simulink model "tqdtqr_rebuild_V3"  (R2021b)
settings: Solver=VariableStepAuto  StartTime=0.0  StopTime=10.0  RelTol=1e-3
undefined symbols (not defined in the file): ATQD_AfterTqMinGain_X_Deg, ATQD_APSCreepBaseTqD_X_kph, ATQD_APSCreepBaseTqD_Y_Deg, ATQD_APSCreepBaseTqR_X_kph, ATQD_APSCreepBaseTqR_Y_Deg, ATQD_APSCreepIterm_X_kph, ATQD_APSCreepIterm_Y_kph, ATQD_APSCreepPterm_X_kph, ATQD_APSCreepPterm_Y_kph, ATQD_APSDecReq_X_kph, ATQD_APSDecReq_Y_mps2, ATQD_APSDecReqCMD_X_kph, ATQD_APSDecReqTs_X_pct, ATQD_APSDecTimeGain_X_Deg, ATQD_APSDecTimeGain_Y_s, ATQD_APSReqLowSpd_X_Deg, ATQD_AutoHoldReleaseBPS_X_Deg, ATQD_AWDLoadTrqnsGain_X_kg, ATQD_AWDLoadTrqnsGain_Y_pct, ATQD_BOSEnBPSPosn_X_kph, ATQD_BOSMap_X_rpm, ATQD_BOSMap_Y_pct, ATQD_CreepBaseTqD_X_kph, ATQD_CreepBaseTqD_Y_Deg, ATQD_CreepBaseTqR_X_kph, ATQD_CreepBaseTqR_Y_Deg, ATQD_CreepBPSDisPosn_X_Deg, ATQD_CreepBPSDisPosnR_X_Deg, ATQD_CreepBPSEnPosn_X_Deg, ATQD_CreepBPSEnPosnR_X_Deg, ATQD_CreepDeltaTq_X_kph, ATQD_CreepIterm_X_kph, ATQD_CreepIterm_Y_kph, ATQD_CreepItermMaxLimit_X_pct, ATQD_CreepPreloadTime_X_kph, ATQD_CreepPreloadTq_X_kph, ATQD_CreepPreloadTq_Y_s, ATQD_CreepProtTq_X_Deg, ATQD_CreepPterm_X_kph, ATQD_CreepPterm_Y_kph, ATQD_CreepRrTqSpRat_X_rpm, ATQD_CreepRrTqSpRat_Y_Nm, ATQD_CreepTargetSpdD_X_pct, ATQD_CreepTargetSpdR_X_pct, ATQD_CreepUpLimitTq_X_rpm, ATQD_DecIneOPDHoldEnDelay_X_Deg, ATQD_DecIneOPDHoldEnDelay_Y_bar, ATQD_ECOTqMapD_X_rpm, ATQD_ECOTqMapD_Y_pct, ATQD_EMTqMapD_X_rpm, ATQD_EMTqMapD_Y_pct, ATQD_EOPDTqMapDCon_X_rpm, ATQD_EOPDTqMapDCon_Y_Deg, ATQD_EstInitVehWeight_X_c, ATQD_FAfterTqCMDGain_X_rpm, ATQD_FAfterTqCMDGain_Y_pct, ATQD_ForceLowSpd_X_Deg, ATQD_ForcePLimitSpd_X_Deg, ATQD_FrLossMAPLowV_X_rpm, ATQD_FrLossMAPLowV_Y_Nm ... (+949)
libraries: simulink x235, hcu_lib x208, tqr x63, tqd x6
(part 1 of 37)
settings Model: Creator=FVT24123  LastModifiedBy=FVT24123

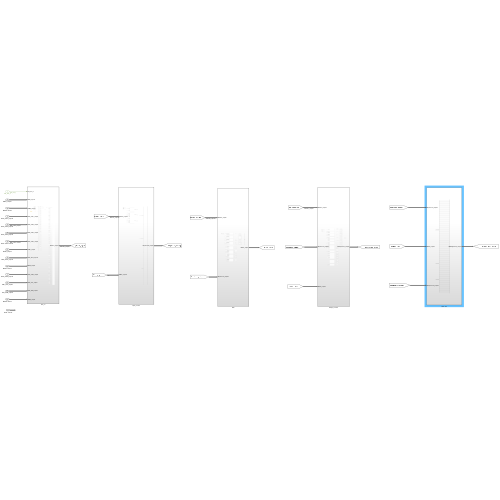
[thumbnail: Simulink's stored preview of the top-level diagram]
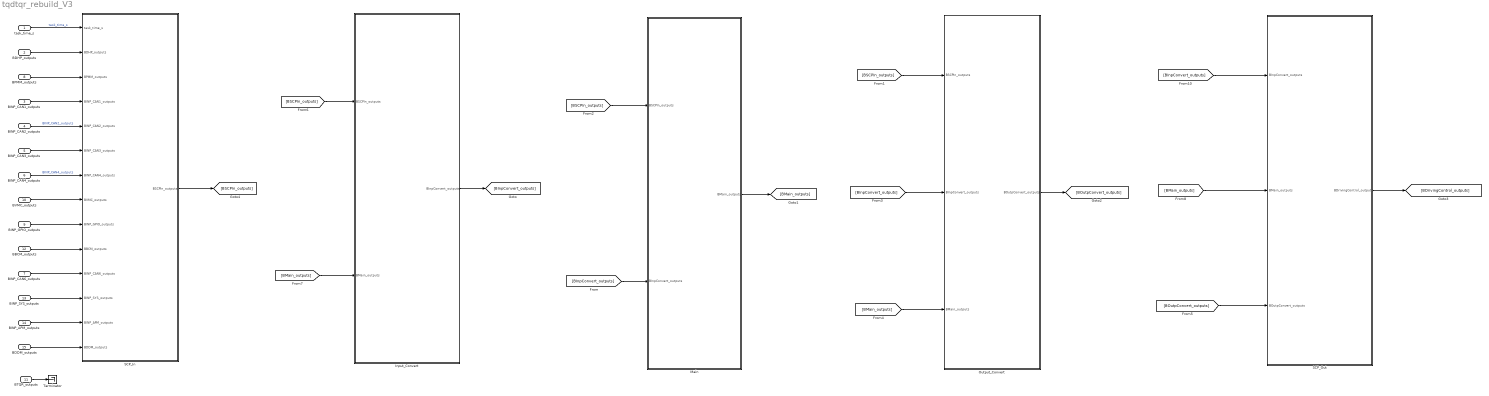
== system tqdtqr_rebuild_V3 ==
  task_time_s : Inport
  BDHP_outputs : Inport  Port=2  OutDataTypeStr=Bus: BDHP_outputs
  BINP_CAN1_outputs : Inport  Port=3  OutDataTypeStr=Bus: BINP_CAN1_outputs
  BINP_CAN2_outputs : Inport  Port=4  OutDataTypeStr=Bus: BINP_CAN2_outputs
  BINP_CAN3_outputs : Inport  Port=5  OutDataTypeStr=Bus: BINP_CAN3_outputs
  BINP_CAN4_outputs : Inport  Port=6  OutDataTypeStr=Bus: BINP_CAN4_outputs
  BINP_CAN6_outputs : Inport  Port=7  OutDataTypeStr=Bus: BINP_CAN6_outputs
  BPMM_outputs : Inport  Port=8  OutDataTypeStr=Bus: BPMM_outputs
  BINP_GPIO_outputs : Inport  Port=9  OutDataTypeStr=Bus: BINP_GPIO_outputs
  BVMC_outputs : Inport  Port=10  OutDataTypeStr=Bus: BVMC_outputs
  BTQR_outputs : Inport  Port=11  OutDataTypeStr=Bus: BTQR_outputs  LockScale=on
  BBCM_outputs : Inport  Port=12  OutDataTypeStr=Bus: BBCM_outputs
  BINP_SYS_outputs : Inport  Port=13  OutDataTypeStr=Bus: BINP_SYS_outputs
  BINP_APM_outputs : Inport  Port=14  OutDataTypeStr=Bus: BINP_APM_outputs
  BDDM_outputs : Inport  Port=15  OutDataTypeStr=Bus: BDDM_outputs
  Input_Convert : Subsystem
  Main : Subsystem
  Output_Convert : Subsystem
  SCP_In : Subsystem
  SCP_Out : Subsystem
  Terminator : Terminator
  wires:
  [BSCPIn_outputs] -> Input_Convert/1(BSCPIn_outputs)
  [BMain_outputs] -> Input_Convert/2(BMain_outputs)
  SCP_In/1(BSCPIn_outputs) -> [BSCPIn_outputs]
  BINP_GPIO_outputs/1 -> SCP_In/9(BINP_GPIO_outputs)
  BTQR_outputs/1 -> Terminator/1
  BINP_SYS_outputs/1 -> SCP_In/12(BINP_SYS_outputs)
  BINP_CAN6_outputs/1 -> SCP_In/11(BINP_CAN6_outputs)
  BDDM_outputs/1 -> SCP_In/14(BDDM_outputs)
  BBCM_outputs/1 -> SCP_In/10(BBCM_outputs)
  BVMC_outputs/1 -> SCP_In/8(BVMC_outputs)
  BDHP_outputs/1 -> SCP_In/2(BDHP_outputs)
  BINP_APM_outputs/1 -> SCP_In/13(BINP_APM_outputs)
  BPMM_outputs/1 -> SCP_In/3(BPMM_outputs)
  BINP_CAN2_outputs/1 -> SCP_In/5(BINP_CAN2_outputs)  "BINP_CAN2_outputs"
  BINP_CAN1_outputs/1 -> SCP_In/4(BINP_CAN1_outputs)
  BINP_CAN4_outputs/1 -> SCP_In/7(BINP_CAN4_outputs)  "BINP_CAN4_outputs"
  task_time_s/1 -> SCP_In/1(task_time_s)  "task_time_s"
  BINP_CAN3_outputs/1 -> SCP_In/6(BINP_CAN3_outputs)
  [BSCPIn_outputs] -> Output_Convert/1(BSCPIn_outputs)
  Input_Convert/1(BInpConvert_outputs) -> [BInpConvert_outputs]
  [BSCPIn_outputs] -> Main/1(BSCPIn_outputs)
  [BInpConvert_outputs] -> Main/2(BInpConvert_outputs)
  Main/1(BMain_outputs) -> [BMain_outputs]
  [BInpConvert_outputs] -> Output_Convert/2(BInpConvert_outputs)
  [BMain_outputs] -> Output_Convert/3(BMain_outputs)
  Output_Convert/1(BOutpConvert_outputs) -> [BOutpConvert_outputs]
  [BInpConvert_outputs] -> SCP_Out/1(BInpConvert_outputs)
  [BMain_outputs] -> SCP_Out/2(BMain_outputs)
  [BOutpConvert_outputs] -> SCP_Out/3(BOutpConvert_outputs)
  SCP_Out/1(BDrivingControl_outputs) -> [BDrivingControl_outputs]

== system tqdtqr_rebuild_V3/Input_Convert ==
  BSCPIn_outputs : Inport
  BMain_outputs : Inport  Port=2
  Bus Creator : BusCreator  Inputs=173
  Bus Selector : BusSelector  OutputSignals=VTQD_LowIdleAccPedal_flg,VTQD_RollRegenDisable_flg,VTQD_BrkSwSta_flg,VTQD_ShiftGearPosn_enum,VTQD_TqTargetShaftSpd_rpm,VTQD_TMRotateDirction_enum,VTQD_EVDriveMode_enum,VTQD_MCUReady4Ext_flg,VTQD_RegenMode_enum,VTQD_FrShaftSpd_rpm,VTQD_RrShaftSpd_rpm,VTQD_LimpHomeAct_flg,VTQD_RDCActive_enum,VTQD_SCPFrRegenAvailTq_Nm,VTQD_SCPRrRegenAvailTq_Nm,VTQD_SCPFrMotorAvailTq_Nm,VTQD_SCPRrMotorAvailTq_Nm,VTQD_SCPFrMCUDCBusVolt_V,VTQD_SCPRrMCUDCBusVolt_V,VTQD_SCPFrMCUTemp_C,VTQD_SCPFrTMTemp_C,VTQD_SCPRrMCUTemp_C,VTQD_SCPRrTMTemp_C,VTQD_SCPSWCRegenUp_flg,VTQD_SCPSWCRegenDown_flg,VTQD_SCPFrEDURotateDirction_enum,VTQD_SCPRrEDURotateDirction_enum,VTQD_SCPFrTMSpd_rpm,VTQD_SCPRrTMSpd_rpm,VTQD_SCPFrEDURealTMTq_Nm,VTQD_SCPRrEDURealTMTq_Nm,VTQD_SCPMCUWarnF_enum,VTQD_SCPMCUWarnR_enum,VTQD_IVIPwrLock_flg,VTQD_IVIPwrLockSta_enum,VTQD_VehActSpd_kph,VTQD_NoSuitbleGear_flg,VTQR_LaunchEn_flg,VTQR_RampTqCMDGain_c,VTQR_EVDriveMode_enum,VTQD_CreepON_flg
  Bus Selector1 : BusSelector  OutputSignals=VTQD_EstVehWeightResult_kg,VTQD_SWCResUpSta_flg,VTQD_SWCSetdownSta_flg,VTQD_SWCCancelSta_flg,SWC_RegenUp,SWC_RegenDown,VTQD_FDCVCURegenMode_enum,VTQD_SaveRegenMode_enum,VTQD_TrailerDisOPDSta_flg,VTQD_SpdCtrlMode_enum,VTQD_SpdCtrlSta_flg,VTQD_SetSpd_kph,VTQD_SWC2ResUpSta_flg,VTQD_SWC2SetdownSta_flg,VTQD_SWC2CancelSta_flg,VTQD_SWC2LADASSta_flg,VTQD_SpdLim4SetSpd_raw32,VTQD_ComboKeyPreEn_flg,VTQD_ComboKeyEn_flg,VTQD_SysMode_enum,VTQD_SWC2ScrollUpSta_flg,VTQD_MaxWhlSlideRate_pct,VTQD_MinWhlSlideRate_pct,VTQD_LeftSlideRate_pct,VTQD_RightSlideRate_pct,VTQD_FrontSlideRate_pct,VTQD_RearSlideRate_pct,VTQD_LFSlideRate_pct,VTQD_LRSlideRate_pct,VTQD_RFSlideRate_pct,VTQD_RRSlideRate_pct,VTQD_SimSouWaveReq_pct,VTQD_SimSoundCmd_pct,VTQD_ActWhlSkipSta_enum,VTQD_SkipDirect_enum,VTQD_GearActualPosn_enum,VTQD_ParkRequest_flg,VTQD_PBWLockTO_flg,VTQD_PBWUnlockTO_flg,VTQD_DriveProtRemove_flg,VTQD_DriveProtEn_flg,VTQD_ForceP_flg,VTQD_DOALatchReq_flg,VTQD_ForcePLimitSpd_kph,VTQD_FrActvDmpDisabReq_flg,VTQD_RrActvDmpDisabReq_flg,VTQD_EPBCarWashMode_flg,VTQD_SWC1SetSpd_kph,VTQD_SWC2SetSpd_kph,VTQD_APSStaSys_enum,VTQD_APSReq_enum,VTQD_APSDecReqA_flg,VTQD_APSDecReq_mps2,VTQD_ActParkRequest_flg,VTQD_APSReqTimer_s,VTQD_OPDHoldEnRel_flg,VTQD_OPDHoldAllowPark_flg,VTQD_OPDHoldLamp_flg,VTQD_OPDHoldActRelTq_Nm,VTQD_OPDHoldDelayForP_flg
  Bus Selector2 : BusSelector  OutputSignals=VTQD_RollRegenEnable_flg,VTQD_BOSEnable_flg,VTQD_BOSTq_Nm,VTQD_IVIRockModeEn_flg,VTQD_LoSpdBrkCtrl_flg,VTQD_RockModeTCSReq_flg,VTQD_RockModePedTq_Nm,VTQD_RockModeTqLim_flg,VTQD_PreLoadPreEn_flg,VTQD_PreloadTq_Nm,VTQD_PreLoadHold_flg,VTQD_CreepWhlTqDem_Nm,VTQD_CreepPrLoadEnable_flg,VTQD_CreepProtTqEn_flg,VTQD_PedalMapWhlTq_Nm,VTQD_EVDriveModeValid_flg,VTQD_RegenTqLimitEn_flg,VTQD_PedAccTqEn_flg,VTQD_SlideRegenLimTq_Nm,VTQD_OPDOn2Off_flg,VTQD_CreepTCSActive_flg,VTQD_FrPreloadTq_Nm,VTQD_RrPreloadTq_Nm,VTQD_CreepEnable_flg,VTQD_CreepBaseTqD_Nm,VTQD_TqSourceFr_enum,VTQD_TqSourceRr_enum,VTQD_TotalWhlTqCapMot_Nm,VTQD_TotalWhlTqCapGen_Nm,VTQD_ForceIdleTqReq_Nm,VTQD_FrEDUSpRat_rat,VTQD_RrEDUSpRat_rat,VTQD_RockModePedTqFr_Nm,VTQD_RockModePedTqRr_Nm,VTQD_TMEnOutpTqSta_enum,VTQD_NewDistFrWhlTq_Nm,VTQD_NewDistRrWhlTq_Nm,VTQD_WhlTqCapMotFr_Nm,VTQD_WhlTqCapMotRr_Nm,VTQD_WhlTqCapGenFr_Nm,VTQD_WhlTqCapGenRr_Nm,VTQD_MotorLossTotal_kW,VTQD_FAfterTqCMDGain_c,VTQD_RAfterTqCMDGain_c,VTQR_FShaftSpdTqLimLow_flg,VTQR_FTimerTqLimLow_flg,VTQR_RShaftSpdTqLimLow_flg,VTQR_RTimerTqLimLow_flg,VTQR_ActFEDUTrqUpLim_Nm,VTQR_ActFEDUTrqLowLim_Nm,VTQR_ActREDUTrqUpLim_Nm,VTQR_ActREDUTrqLowLim_Nm,VTQR_FrTqZeroTransUpBound_Nm,VTQR_FrTqZeroTransLowBound_Nm,VTQR_FrTqZeroTrans_enum,VTQR_RrTqZeroTransUpBound_Nm,VTQR_RrTqZeroTransLowBound_Nm,VTQR_RrTqZeroTrans_enum,VTQR_FrGearChange_flg,VTQR_RrGearChange_flg,VTQR_FrFirstOrderInpTs_c,VTQR_FrRateLimitInc_Nm,VTQR_FrRateLimitDec_Nm,VTQR_RrFirstOrderInpTs_c,VTQR_RrRateLimitInc_Nm,VTQR_RrRateLimitDec_Nm,VTQD_FEDUWhlTqBRegen_Nm,VTQD_REDUWhlTqBRegen_Nm,VTQR_ActFEDUTqLowLimit_Nm,VTQR_ActFEDUTqUpLimit_Nm,VTQR_ActREDUTqUpLimit_Nm,VTQR_ActREDUTqLowLimit_Nm
  Input Signal Convert : Subsystem
  Main function : Subsystem
  Signal function : Subsystem
  BInpConvert_outputs : Outport
  wires:
  BSCPIn_outputs/1 -> [BSCPIn_outputs]
  [BSCPIn_outputs] -> Input Signal Convert/1(BSCPIn_outputs)
  [BSCPIn_outputs] -> Signal function/1(BSCPIn_outputs)
  Input Signal Convert/1(BSignalConvert_outputs) -> [BSignalConvert_outputs]
  [BSignalConvert_outputs] -> Signal function/2(BSignalConvert_outputs)
  [BMain_outputs] -> Signal function/3(BMain_outputs)
  BMain_outputs/1 -> [BMain_outputs]
  [BFunction_outputs] -> Input Signal Convert/2(BFunction_outputs)
  Signal function/1(BFunction_outputs) -> [BFunction_outputs]
  Bus Selector/1 -> Bus Creator/1  "<VTQD_LowIdleAccPedal_flg>"
  Bus Selector/2 -> Bus Creator/2  "<VTQD_RollRegenDisable_flg>"
  Bus Selector/3 -> Bus Creator/3  "<VTQD_BrkSwSta_flg>"
  Bus Selector/4 -> Bus Creator/4  "<VTQD_ShiftGearPosn_enum>"
  Bus Selector/5 -> Bus Creator/5  "<VTQD_TqTargetShaftSpd_rpm>"
  Bus Selector/6 -> Bus Creator/6  "<VTQD_TMRotateDirction_enum>"
  Bus Selector/7 -> Bus Creator/7  "<VTQD_EVDriveMode_enum>"
  Bus Selector/8 -> Bus Creator/8  "<VTQD_MCUReady4Ext_flg>"
  Bus Selector/9 -> Bus Creator/9  "<VTQD_RegenMode_enum>"
  Bus Selector/10 -> Bus Creator/10  "<VTQD_FrShaftSpd_rpm>"
  Bus Selector/11 -> Bus Creator/11  "<VTQD_RrShaftSpd_rpm>"
  Bus Selector/12 -> Bus Creator/12  "<VTQD_LimpHomeAct_flg>"
  Bus Selector/13 -> Bus Creator/13  "<VTQD_RDCActive_enum>"
  Bus Selector/14 -> Bus Creator/14  "<VTQD_SCPFrRegenAvailTq_Nm>"
  Bus Selector/15 -> Bus Creator/15  "<VTQD_SCPRrRegenAvailTq_Nm>"
  Bus Selector/16 -> Bus Creator/16  "<VTQD_SCPFrMotorAvailTq_Nm>"
  Bus Selector/17 -> Bus Creator/17  "<VTQD_SCPRrMotorAvailTq_Nm>"
  Bus Selector/18 -> Bus Creator/18  "<VTQD_SCPFrMCUDCBusVolt_V>"
  [BFunction_outputs] -> Bus Selector1/1
  Bus Selector/19 -> Bus Creator/19  "<VTQD_SCPRrMCUDCBusVolt_V>"
  Bus Selector/20 -> Bus Creator/20  "<VTQD_SCPFrMCUTemp_C>"
  Bus Selector/21 -> Bus Creator/21  "<VTQD_SCPFrTMTemp_C>"
  Bus Selector/22 -> Bus Creator/22  "<VTQD_SCPRrMCUTemp_C>"
  Bus Selector/23 -> Bus Creator/23  "<VTQD_SCPRrTMTemp_C>"
  Bus Selector/24 -> Bus Creator/24  "<VTQD_SCPSWCRegenUp_flg>"
  Bus Selector/25 -> Bus Creator/25  "<VTQD_SCPSWCRegenDown_flg>"
  Bus Selector/26 -> Bus Creator/26  "<VTQD_SCPFrEDURotateDirction_enum>"
  Bus Selector/27 -> Bus Creator/27  "<VTQD_SCPRrEDURotateDirction_enum>"
  Bus Selector/28 -> Bus Creator/28  "<VTQD_SCPFrTMSpd_rpm>"
  Bus Selector/29 -> Bus Creator/29  "<VTQD_SCPRrTMSpd_rpm>"
  Bus Selector/30 -> Bus Creator/30  "<VTQD_SCPFrEDURealTMTq_Nm>"
  Bus Selector/31 -> Bus Creator/31  "<VTQD_SCPRrEDURealTMTq_Nm>"
  Bus Selector/32 -> Bus Creator/32  "<VTQD_SCPMCUWarnF_enum>"
  Bus Selector/33 -> Bus Creator/33  "<VTQD_SCPMCUWarnR_enum>"
  Bus Selector1/1 -> Bus Creator/42  "<VTQD_EstVehWeightResult_kg>"
  Bus Selector1/2 -> Bus Creator/43  "<VTQD_SWCResUpSta_flg>"
  Bus Selector1/3 -> Bus Creator/44  "<VTQD_SWCSetdownSta_flg>"
  Bus Selector1/4 -> Bus Creator/45  "<VTQD_SWCCancelSta_flg>"
  Bus Selector1/5 -> Bus Creator/46  "<SWC_RegenUp>"
  Bus Selector1/6 -> Bus Creator/47  "<SWC_RegenDown>"
  Bus Selector1/7 -> Bus Creator/48  "<VTQD_FDCVCURegenMode_enum>"
  Bus Selector1/8 -> Bus Creator/49  "<VTQD_SaveRegenMode_enum>"
  Bus Selector1/9 -> Bus Creator/50  "<VTQD_TrailerDisOPDSta_flg>"
  Bus Selector1/10 -> Bus Creator/51  "<VTQD_SpdCtrlMode_enum>"
  Bus Selector1/11 -> Bus Creator/52  "<VTQD_SpdCtrlSta_flg>"
  Bus Selector1/12 -> Bus Creator/53  "<VTQD_SetSpd_kph>"
  Bus Selector1/13 -> Bus Creator/54  "<VTQD_SWC2ResUpSta_flg>"
  Bus Selector1/14 -> Bus Creator/55  "<VTQD_SWC2SetdownSta_flg>"
  Bus Selector1/15 -> Bus Creator/56  "<VTQD_SWC2CancelSta_flg>"
  Bus Selector1/16 -> Bus Creator/57  "<VTQD_SWC2LADASSta_flg>"
  Bus Selector1/17 -> Bus Creator/58  "<VTQD_SpdLim4SetSpd_raw32>"
  Bus Selector1/18 -> Bus Creator/59  "<VTQD_ComboKeyPreEn_flg>"
  Bus Selector1/19 -> Bus Creator/60  "<VTQD_ComboKeyEn_flg>"
  Bus Selector1/20 -> Bus Creator/61  "<VTQD_SysMode_enum>"
  Bus Creator/1 -> BInpConvert_outputs/1
  [BSignalConvert_outputs] -> Bus Selector/1
  Bus Selector1/48 -> Bus Creator/89  "<VTQD_SWC1SetSpd_kph>"
  Bus Selector1/49 -> Bus Creator/90  "<VTQD_SWC2SetSpd_kph>"
  [DriverWhlTqDemFunc_outputs] -> Bus Selector2/1
  Bus Selector2/1 -> Bus Creator/102  "<VTQD_RollRegenEnable_flg>"
  Bus Selector2/2 -> Bus Creator/103  "<VTQD_BOSEnable_flg>"
  Bus Selector2/3 -> Bus Creator/104  "<VTQD_BOSTq_Nm>"
  Bus Selector2/5 -> Bus Creator/106  "<VTQD_LoSpdBrkCtrl_flg>"
  Bus Selector2/7 -> Bus Creator/108  "<VTQD_RockModePedTq_Nm>"
  Bus Selector2/8 -> Bus Creator/109  "<VTQD_RockModeTqLim_flg>"
  Bus Selector2/9 -> Bus Creator/110  "<VTQD_PreLoadPreEn_flg>"
  Bus Selector2/10 -> Bus Creator/111  "<VTQD_PreloadTq_Nm>"
  Bus Selector2/11 -> Bus Creator/112  "<VTQD_PreLoadHold_flg>"
  Bus Selector2/12 -> Bus Creator/113  "<VTQD_CreepWhlTqDem_Nm>"
  Bus Selector2/13 -> Bus Creator/114  "<VTQD_CreepPrLoadEnable_flg>"
  Bus Selector2/14 -> Bus Creator/115  "<VTQD_CreepProtTqEn_flg>"
  Bus Selector2/15 -> Bus Creator/116  "<VTQD_PedalMapWhlTq_Nm>"
  Bus Selector2/16 -> Bus Creator/117  "<VTQD_EVDriveModeValid_flg>"
  Bus Selector2/17 -> Bus Creator/118  "<VTQD_RegenTqLimitEn_flg>"
  Bus Selector2/18 -> Bus Creator/119  "<VTQD_PedAccTqEn_flg>"
  Bus Selector2/19 -> Bus Creator/120  "<VTQD_SlideRegenLimTq_Nm>"
  Bus Selector2/20 -> Bus Creator/121  "<VTQD_OPDOn2Off_flg>"
  Bus Selector2/21 -> Bus Creator/122  "<VTQD_CreepTCSActive_flg>"
  Bus Selector2/22 -> Bus Creator/123  "<VTQD_FrPreloadTq_Nm>"
  Bus Selector/36 -> Bus Creator/36  "<VTQD_VehActSpd_kph>"
  Bus Selector2/23 -> Bus Creator/124  "<VTQD_RrPreloadTq_Nm>"
  Bus Selector2/24 -> Bus Creator/125  "<VTQD_CreepEnable_flg>"
  Bus Selector2/25 -> Bus Creator/126  "<VTQD_CreepBaseTqD_Nm>"
  [BMain_outputs] -> Main function/4(BMain_outputs)
  [BSignalConvert_outputs] -> Main function/2(BSignalConvert_outputs)
  [BSCPIn_outputs] -> Main function/1(BSCPIn_outputs)
  [BFunction_outputs] -> Main function/3(BFunction_outputs)
  Main function/1(MainFunction_outputs) -> [DriverWhlTqDemFunc_outputs]
  Bus Selector/37 -> Bus Creator/37  "<VTQD_NoSuitbleGear_flg>"
  [DriverWhlTqDemFunc_outputs] -> Signal function/4(DriverWhlTqDemFunc_outputs)
  Bus Selector2/4 -> Bus Creator/105  "<VTQD_IVIRockModeEn_flg>"
  Bus Selector2/6 -> Bus Creator/107  "<VTQD_RockModeTCSReq_flg>"
  Bus Selector1/21 -> Bus Creator/62  "<VTQD_SWC2ScrollUpSta_flg>"
  Bus Selector1/22 -> Bus Creator/63  "<VTQD_MaxWhlSlideRate_pct>"
  Bus Selector1/23 -> Bus Creator/64  "<VTQD_MinWhlSlideRate_pct>"
  Bus Selector1/24 -> Bus Creator/65  "<VTQD_LeftSlideRate_pct>"
  Bus Selector1/25 -> Bus Creator/66  "<VTQD_RightSlideRate_pct>"
  Bus Selector1/26 -> Bus Creator/67  "<VTQD_FrontSlideRate_pct>"
  Bus Selector1/27 -> Bus Creator/68  "<VTQD_RearSlideRate_pct>"
  Bus Selector1/28 -> Bus Creator/69  "<VTQD_LFSlideRate_pct>"
  Bus Selector1/29 -> Bus Creator/70  "<VTQD_LRSlideRate_pct>"
  Bus Selector1/30 -> Bus Creator/71  "<VTQD_RFSlideRate_pct>"
  Bus Selector1/31 -> Bus Creator/72  "<VTQD_RRSlideRate_pct>"
  Bus Selector1/32 -> Bus Creator/73  "<VTQD_SimSouWaveReq_pct>"
  Bus Selector1/33 -> Bus Creator/74  "<VTQD_SimSoundCmd_pct>"
  Bus Selector1/34 -> Bus Creator/75  "<VTQD_ActWhlSkipSta_enum>"
  Bus Selector1/35 -> Bus Creator/76  "<VTQD_SkipDirect_enum>"
  Bus Selector1/36 -> Bus Creator/77  "<VTQD_GearActualPosn_enum>"
  Bus Selector1/37 -> Bus Creator/78  "<VTQD_ParkRequest_flg>"
  Bus Selector1/38 -> Bus Creator/79  "<VTQD_PBWLockTO_flg>"
  Bus Selector1/39 -> Bus Creator/80  "<VTQD_PBWUnlockTO_flg>"
  Bus Selector1/40 -> Bus Creator/81  "<VTQD_DriveProtRemove_flg>"
  Bus Selector1/41 -> Bus Creator/82  "<VTQD_DriveProtEn_flg>"
  Bus Selector1/42 -> Bus Creator/83  "<VTQD_ForceP_flg>"
  Bus Selector1/45 -> Bus Creator/86  "<VTQD_FrActvDmpDisabReq_flg>"
  Bus Selector1/46 -> Bus Creator/87  "<VTQD_RrActvDmpDisabReq_flg>"
  Bus Selector1/47 -> Bus Creator/88  "<VTQD_EPBCarWashMode_flg>"
  Bus Selector/34 -> Bus Creator/34  "<VTQD_IVIPwrLock_flg>"
  Bus Selector/35 -> Bus Creator/35  "<VTQD_IVIPwrLockSta_enum>"
  Bus Selector1/60 -> Bus Creator/101  "<VTQD_OPDHoldDelayForP_flg>"
  Bus Selector1/59 -> Bus Creator/100  "<VTQD_OPDHoldActRelTq_Nm>"
  Bus Selector1/58 -> Bus Creator/99  "<VTQD_OPDHoldLamp_flg>"
  Bus Selector1/57 -> Bus Creator/98  "<VTQD_OPDHoldAllowPark_flg>"
  Bus Selector1/56 -> Bus Creator/97  "<VTQD_OPDHoldEnRel_flg>"
  Bus Selector1/55 -> Bus Creator/96  "<VTQD_APSReqTimer_s>"
  Bus Selector1/54 -> Bus Creator/95  "<VTQD_ActParkRequest_flg>"
  Bus Selector1/53 -> Bus Creator/94  "<VTQD_APSDecReq_mps2>"
  Bus Selector1/52 -> Bus Creator/93  "<VTQD_APSDecReqA_flg>"
  Bus Selector1/51 -> Bus Creator/92  "<VTQD_APSReq_enum>"
  Bus Selector1/50 -> Bus Creator/91  "<VTQD_APSStaSys_enum>"
  Bus Selector/38 -> Bus Creator/38  "<VTQR_LaunchEn_flg>"
  Bus Selector/39 -> Bus Creator/39  "<VTQR_RampTqCMDGain_c>"
  Bus Selector/40 -> Bus Creator/40  "<VTQR_EVDriveMode_enum>"
  Bus Selector2/26 -> Bus Creator/127  "<VTQD_TqSourceFr_enum>"
  Bus Selector2/27 -> Bus Creator/128  "<VTQD_TqSourceRr_enum>"
  Bus Selector2/28 -> Bus Creator/129  "<VTQD_TotalWhlTqCapMot_Nm>"
  Bus Selector2/29 -> Bus Creator/130  "<VTQD_TotalWhlTqCapGen_Nm>"
  Bus Selector2/38 -> Bus Creator/139  "<VTQD_WhlTqCapMotFr_Nm>"
  Bus Selector2/39 -> Bus Creator/140  "<VTQD_WhlTqCapMotRr_Nm>"
  Bus Selector2/40 -> Bus Creator/141  "<VTQD_WhlTqCapGenFr_Nm>"
  Bus Selector2/41 -> Bus Creator/142  "<VTQD_WhlTqCapGenRr_Nm>"
  Bus Selector2/42 -> Bus Creator/143  "<VTQD_MotorLossTotal_kW>"
  Bus Selector2/43 -> Bus Creator/144  "<VTQD_FAfterTqCMDGain_c>"
  Bus Selector2/44 -> Bus Creator/145  "<VTQD_RAfterTqCMDGain_c>"
  Bus Selector2/45 -> Bus Creator/146  "<VTQR_FShaftSpdTqLimLow_flg>"
  Bus Selector2/46 -> Bus Creator/147  "<VTQR_FTimerTqLimLow_flg>"
  Bus Selector2/47 -> Bus Creator/148  "<VTQR_RShaftSpdTqLimLow_flg>"
  Bus Selector2/48 -> Bus Creator/149  "<VTQR_RTimerTqLimLow_flg>"
  Bus Selector2/49 -> Bus Creator/150  "<VTQR_ActFEDUTrqUpLim_Nm>"
  Bus Selector2/50 -> Bus Creator/151  "<VTQR_ActFEDUTrqLowLim_Nm>"
  Bus Selector2/51 -> Bus Creator/152  "<VTQR_ActREDUTrqUpLim_Nm>"
  Bus Selector2/52 -> Bus Creator/153  "<VTQR_ActREDUTrqLowLim_Nm>"
  Bus Selector2/53 -> Bus Creator/154  "<VTQR_FrTqZeroTransUpBound_Nm>"
  Bus Selector2/54 -> Bus Creator/155  "<VTQR_FrTqZeroTransLowBound_Nm>"
  Bus Selector2/55 -> Bus Creator/156  "<VTQR_FrTqZeroTrans_enum>"
  Bus Selector2/56 -> Bus Creator/157  "<VTQR_RrTqZeroTransUpBound_Nm>"
  Bus Selector2/57 -> Bus Creator/158  "<VTQR_RrTqZeroTransLowBound_Nm>"
  Bus Selector2/58 -> Bus Creator/159  "<VTQR_RrTqZeroTrans_enum>"
  Bus Selector2/59 -> Bus Creator/160  "<VTQR_FrGearChange_flg>"
  Bus Selector2/60 -> Bus Creator/161  "<VTQR_RrGearChange_flg>"
  Bus Selector2/61 -> Bus Creator/162  "<VTQR_FrFirstOrderInpTs_c>"
  Bus Selector2/62 -> Bus Creator/163  "<VTQR_FrRateLimitInc_Nm>"
  Bus Selector2/63 -> Bus Creator/164  "<VTQR_FrRateLimitDec_Nm>"
  Bus Selector2/64 -> Bus Creator/165  "<VTQR_RrFirstOrderInpTs_c>"
  Bus Selector2/65 -> Bus Creator/166  "<VTQR_RrRateLimitInc_Nm>"
  Bus Selector2/66 -> Bus Creator/167  "<VTQR_RrRateLimitDec_Nm>"
  Bus Selector2/67 -> Bus Creator/168  "<VTQD_FEDUWhlTqBRegen_Nm>"
  Bus Selector2/68 -> Bus Creator/169  "<VTQD_REDUWhlTqBRegen_Nm>"
  Bus Selector2/69 -> Bus Creator/170  "<VTQR_ActFEDUTqLowLimit_Nm>"
  Bus Selector2/70 -> Bus Creator/171  "<VTQR_ActFEDUTqUpLimit_Nm>"
  Bus Selector2/71 -> Bus Creator/172  "<VTQR_ActREDUTqUpLimit_Nm>"
  Bus Selector2/72 -> Bus Creator/173  "<VTQR_ActREDUTqLowLimit_Nm>"
  [BMain_outputs] -> Input Signal Convert/3(BMain_outputs)
  Bus Selector1/43 -> Bus Creator/84  "<VTQD_DOALatchReq_flg>"
  Bus Selector1/44 -> Bus Creator/85  "<VTQD_ForcePLimitSpd_kph>"
  Bus Selector2/30 -> Bus Creator/131  "<VTQD_ForceIdleTqReq_Nm>"
  Bus Selector2/31 -> Bus Creator/132  "<VTQD_FrEDUSpRat_rat>"
  Bus Selector2/32 -> Bus Creator/133  "<VTQD_RrEDUSpRat_rat>"
  Bus Selector2/33 -> Bus Creator/134  "<VTQD_RockModePedTqFr_Nm>"
  Bus Selector2/34 -> Bus Creator/135  "<VTQD_RockModePedTqRr_Nm>"
  Bus Selector2/35 -> Bus Creator/136  "<VTQD_TMEnOutpTqSta_enum>"
  Bus Selector2/36 -> Bus Creator/137  "<VTQD_NewDistFrWhlTq_Nm>"
  Bus Selector2/37 -> Bus Creator/138  "<VTQD_NewDistRrWhlTq_Nm>"
  Bus Selector/41 -> Bus Creator/41  "<VTQD_CreepON_flg>"

== system tqdtqr_rebuild_V3/Main ==
  note: --------------------------------------------------------------------TQR-----------------------------------------------------------------------
  BSCPIn_outputs : Inport
  BInpConvert_outputs : Inport  Port=2
  Avaliable Tq Limit : Subsystem
  Bus Creator : BusCreator  Inputs=22
  DriverWhlTqDem : Subsystem
  Front/Rear final torque : Subsystem
  Front/Rear first order input torque : Subsystem
  Front/Rear ramp enable judge : Subsystem
  Inverse and turn to motor torque : Subsystem
  Tq Coordination : Subsystem
  Tq Distribution : Subsystem
  BMain_outputs : Outport
  wires:
  BSCPIn_outputs/1 -> [BSCPIn_outputs]
  BInpConvert_outputs/1 -> [BInpConvert_outputs]
  [BSCPIn_outputs] -> DriverWhlTqDem/1(BSCPIn_outputs)
  [BInpConvert_outputs] -> DriverWhlTqDem/2(BInpConvert_outputs)
  DriverWhlTqDem/1(VTQD_DriverWhlTqDem_Nm) -> [VTQD_DriverWhlTqDem_Nm]
  [BSCPIn_outputs] -> Tq Coordination/1(BSCPIn_outputs)
  [BInpConvert_outputs] -> Tq Coordination/2(BInpConvert_outputs)
  [VTQD_DriverWhlTqDem_Nm] -> Tq Coordination/3(VTQD_DriverWhlTqDem_Nm)
  [BSCPIn_outputs] -> Tq Distribution/1(BSCPIn_outputs)
  [BInpConvert_outputs] -> Tq Distribution/2(BInpConvert_outputs)
  Tq Coordination/1(VTQD_CoordTqDem_Nm) -> [VTQD_CoordTqDem_Nm]
  [VTQD_CoordTqDem_Nm] -> Tq Distribution/3(TqCoordination_outputs)
  Tq Distribution/1(VTQD_CoordWhlTqDemFr_Nm) -> [VTQD_CoordWhlTqDemFr_Nm]
  [VTQD_DriverWhlTqDem_Nm] -> Bus Creator/1
  [VTQD_CoordTqDem_Nm] -> Bus Creator/2
  Bus Creator/1 -> BMain_outputs/1
  Tq Distribution/2(VTQD_CoordWhlTqDemRr_Nm) -> [VTQD_CoordWhlTqDemRr_Nm]
  [VTQD_CoordWhlTqDemFr_Nm] -> Bus Creator/3
  [BInpConvert_outputs] -> Avaliable Tq Limit/2(BInpConvert_outputs)
  [BSCPIn_outputs] -> Avaliable Tq Limit/1(BSCPIn_outputs)
  [VTQD_CoordWhlTqDemFr_Nm] -> Avaliable Tq Limit/3(VTQD_CoordWhlTqDemFr_Nm)
  [VTQD_CoordWhlTqDemRr_Nm] -> Avaliable Tq Limit/4(VTQD_CoordWhlTqDemRr_Nm)
  Avaliable Tq Limit/2(VTQD_AfterAvailableTqDemRr_Nm) -> [VTQD_AfterAvailableTqDemRr_Nm]
  Avaliable Tq Limit/1(VTQD_AfterAvailableTqDemFr_Nm) -> [VTQD_AfterAvailableTqDemFr_Nm]
  [VTQD_AfterAvailableTqDemFr_Nm] -> Bus Creator/7
  [VTQD_AfterAvailableTqDemRr_Nm] -> Bus Creator/8
  [BInpConvert_outputs] -> Front/Rear first order input torque/1(BInpConvert_outputs)
  [VTQD_AfterAvailableTqDemFr_Nm] -> Front/Rear first order input torque/2(VTQD_AfterAvailableTqDemFr_Nm)
  [VTQD_AfterAvailableTqDemRr_Nm] -> Front/Rear first order input torque/3(VTQD_AfterAvailableTqDemRr_Nm)
  Front/Rear first order input torque/1(VTQR_FrFirstOrderInpTq_Nm) -> [VTQR_FrFirstOrderInpTq_Nm]
  Front/Rear first order input torque/2(VTQR_RrFirstOrderInpTq_Nm) -> [VTQR_RrFirstOrderInpTq_Nm]
  [BInpConvert_outputs] -> Front/Rear final torque/2(BInpConvert_outputs)
  [VTQR_FrFirstOrderInpTq_Nm] -> Front/Rear final torque/3(VTQR_FrFirstOrderInpTq_Nm)
  [VTQR_RrFirstOrderInpTq_Nm] -> Front/Rear final torque/4(VTQR_RrFirstOrderInpTq_Nm)
  [BSCPIn_outputs] -> Front/Rear final torque/1(BSCPIn_outputs)
  Front/Rear final torque/1(VTQR_FrFirstOrderOutTqDelay_Nm) -> [VTQR_FrFirstOrderOutTqDelay_Nm]
  Front/Rear final torque/2(VTQR_FEDUWhlTqReqSmoothDelay_Nm) -> [VTQR_FEDUWhlTqReqSmoothDelay_Nm]
  Front/Rear final torque/3(VTQR_RampFEDUWhlTqReq_Nm) -> [VTQR_RampFEDUWhlTqReq_Nm]
  Front/Rear final torque/4(VTQR_RrFirstOrderOutTqDelay_Nm) -> [VTQR_RrFirstOrderOutTqDelay_Nm]
  Front/Rear final torque/5(VTQR_REDUWhlTqReqSmoothDelay_Nm) -> [VTQR_REDUWhlTqReqSmoothDelay_Nm]
  Front/Rear final torque/6(VTQR_RampREDUWhlTqReq_Nm) -> [VTQR_RampREDUWhlTqReq_Nm]
  [VTQR_FrFirstOrderOutTqDelay_Nm] -> Bus Creator/11
  [VTQR_FEDUWhlTqReqSmoothDelay_Nm] -> Bus Creator/12
  [VTQR_RampFEDUWhlTqReq_Nm] -> Bus Creator/13
  [VTQR_RrFirstOrderOutTqDelay_Nm] -> Bus Creator/14
  [VTQR_REDUWhlTqReqSmoothDelay_Nm] -> Bus Creator/15
  [VTQR_RampREDUWhlTqReq_Nm] -> Bus Creator/16
  [VTQR_FrFirstOrderInpTq_Nm] -> Bus Creator/9
  [VTQR_RrFirstOrderInpTq_Nm] -> Bus Creator/10
  [VTQR_FrFirstOrderOutTqDelay_Nm] -> Front/Rear first order input torque/4(VTQR_FrFirstOrderOutTqDelay_Nm)
  [VTQR_RrFirstOrderOutTqDelay_Nm] -> Front/Rear first order input torque/5(VTQR_RrFirstOrderOutTqDelay_Nm)
  [BSCPIn_outputs] -> Front/Rear ramp enable judge/1(BSCPIn_outputs)
  [BInpConvert_outputs] -> Front/Rear ramp enable judge/2(BInpConvert_outputs)
  [VTQR_RampFEDUWhlTqReq_Nm] -> Front/Rear ramp enable judge/3(VTQR_RampFEDUWhlTqReq_Nm)
  [VTQD_AfterAvailableTqDemFr_Nm] -> Front/Rear ramp enable judge/4(VTQD_AfterAvailableTqDemFr_Nm)
  [VTQR_RampREDUWhlTqReq_Nm] -> Front/Rear ramp enable judge/5(VTQR_RampREDUWhlTqReq_Nm)
  [VTQD_AfterAvailableTqDemRr_Nm] -> Front/Rear ramp enable judge/6(VTQD_AfterAvailableTqDemRr_Nm)
  Front/Rear ramp enable judge/1(VTQR_ActualFEDUWhlTqReq_Nm) -> [VTQR_ActualFEDUWhlTqReq_Nm]
  Front/Rear ramp enable judge/2(VTQR_NoABSFEDUWhlTqReq_Nm) -> [VTQR_NoABSFEDUWhlTqReq_Nm]
  Front/Rear ramp enable judge/3(VTQR_ActualREDUWhlTqReq_Nm) -> [VTQR_ActualREDUWhlTqReq_Nm]
  Front/Rear ramp enable judge/4(VTQR_NoABSREDUWhlTqReq_Nm) -> [VTQR_NoABSREDUWhlTqReq_Nm]
  [VTQR_ActualFEDUWhlTqReq_Nm] -> Bus Creator/17
  [VTQR_NoABSFEDUWhlTqReq_Nm] -> Bus Creator/18
  [VTQR_ActualREDUWhlTqReq_Nm] -> Bus Creator/19
  [VTQR_NoABSREDUWhlTqReq_Nm] -> Bus Creator/20
  [BSCPIn_outputs] -> Inverse and turn to motor torque/1(BSCPIn_outputs)
  [BInpConvert_outputs] -> Inverse and turn to motor torque/2(BInpConvert_outputs)
  [VTQR_ActualFEDUWhlTqReq_Nm] -> Inverse and turn to motor torque/3(VTQR_ActualFEDUWhlTqReq_Nm)
  [VTQR_ActualREDUWhlTqReq_Nm] -> Inverse and turn to motor torque/4(VTQR_ActualREDUWhlTqReq_Nm)
  Inverse and turn to motor torque/1(VTQR_FrTMTqReq_Nm) -> [VTQR_FrTMTqReq_Nm]
  Inverse and turn to motor torque/2(VTQR_RrTMTqReq_Nm) -> [VTQR_RrTMTqReq_Nm]
  [VTQR_FrTMTqReq_Nm] -> Bus Creator/21
  [VTQR_RrTMTqReq_Nm] -> Bus Creator/22
  Tq Distribution/3(VTQD_CoordTqDemFr_Nm) -> [VTQD_CoordTqDemFr_Nm]
  Tq Distribution/4(VTQD_CoordTqDemRr_Nm) -> [VTQD_CoordTqDemRr_Nm]
  [VTQD_CoordWhlTqDemRr_Nm] -> Bus Creator/4
  [VTQD_CoordTqDemFr_Nm] -> Bus Creator/5
  [VTQD_CoordTqDemRr_Nm] -> Bus Creator/6

== system tqdtqr_rebuild_V3/Output_Convert ==
  BSCPIn_outputs : Inport
  BInpConvert_outputs : Inport  Port=2
  BMain_outputs : Inport  Port=3
  Avaliable Torque : Subsystem
  Bus Creator : BusCreator  Inputs=45
  CrashDetect : Subsystem
  ESC/TCS demand torque : Subsystem
  Equivalent Acceleration Pedal Switch signal : Subsystem
  ExtTqFuncHandShaking : Subsystem
  P_Button_State_Judge : Subsystem
  Regen Limited Indicator signal : Subsystem
  SWC1 SWC2 set speed warning : Subsystem
  Signal for ESC : Subsystem
  Signals for BCM : Subsystem
  Signals for MCU : Subsystem
  BOutpConvert_outputs : Outport
  wires:
  BSCPIn_outputs/1 -> [BSCPIn_outputs]
  [BMain_outputs] -> Equivalent Acceleration Pedal Switch signal/3(BMain_outputs)
  BInpConvert_outputs/1 -> [BInpConvert_outputs]
  Equivalent Acceleration Pedal Switch signal/1(VTQD_EquivAccPedalSWSta_flg) -> [VTQD_EquivAccPedalSWSta_flg]
  Regen Limited Indicator signal/1(VTQD_RegenLimIndSta_flg) -> [VTQD_RegenLimIndSta_flg]
  [VTQD_CrashDetd_flg] -> Bus Creator/1
  [VTQD_DiagHCrash_flg] -> Bus Creator/2
  [VTQD_EquivAccPedalSWSta_flg] -> Bus Creator/5
  [VTQD_RegenLimIndSta_flg] -> Bus Creator/6
  Bus Creator/1 -> BOutpConvert_outputs/1
  SWC1 SWC2 set speed warning/1(VTQD_SetSpdLimWarn_flg) -> [VTQD_SetSpdLimWarn_flg]
  [VTQD_SetSpdLimWarn_flg] -> Bus Creator/7
  P_Button_State_Judge/1(VTQD_PButtonSta_enum) -> [VTQD_PButtonSta_enum]
  [VTQD_PButtonSta_enum] -> Bus Creator/8
  [BSCPIn_outputs] -> Equivalent Acceleration Pedal Switch signal/1(BSCPIn_outputs)
  [BInpConvert_outputs] -> Equivalent Acceleration Pedal Switch signal/2(BInpConvert_outputs)
  [BInpConvert_outputs] -> Regen Limited Indicator signal/2(BInpConvert_outputs)
  [BSCPIn_outputs] -> Regen Limited Indicator signal/1(BSCPIn_outputs)
  [BSCPIn_outputs] -> SWC1 SWC2 set speed warning/1(BSCPIn_outputs)
  [BInpConvert_outputs] -> SWC1 SWC2 set speed warning/2(BInpConvert_outputs)
  [BSCPIn_outputs] -> P_Button_State_Judge/1(BSCPIn_outputs)
  [BInpConvert_outputs] -> P_Button_State_Judge/2(BInpConvert_outputs)
  BMain_outputs/1 -> [BMain_outputs]
  [BMain_outputs] -> Regen Limited Indicator signal/3(BMain_outputs)
  [BSCPIn_outputs] -> ESC/TCS demand torque/1(BSCPIn_outputs)
  [BInpConvert_outputs] -> ESC/TCS demand torque/2(BInpConvert_outputs)
  [BMain_outputs] -> ESC/TCS demand torque/3(BMain_outputs)
  ESC/TCS demand torque/1(VTQD_DriverWhlTqDemFr_Nm) -> [VTQD_DriverWhlTqDemFr_Nm]
  ESC/TCS demand torque/2(VTQD_DriverWhlTqDemRr_Nm) -> [VTQD_DriverWhlTqDemRr_Nm]
  [BSCPIn_outputs] -> Avaliable Torque/1(BSCPIn_outputs)
  [BInpConvert_outputs] -> Avaliable Torque/2(BInpConvert_outputs)
  [BMain_outputs] -> Avaliable Torque/3(BMain_outputs)
  [VTQD_DriverWhlTqDemFr_Nm] -> Avaliable Torque/4(VTQD_DriverWhlTqDemFr_Nm)
  [VTQD_DriverWhlTqDemRr_Nm] -> Avaliable Torque/5(VTQD_DriverWhlTqDemRr_Nm)
  Avaliable Torque/1(VTQD_ARegenActive_flg) -> [VTQD_ARegenActive_flg]
  Avaliable Torque/2(VTQD_FrEDUAvailBrkRgnTq_Nm) -> [VTQD_FrEDUAvailBrkRgnTq_Nm]
  Avaliable Torque/3(VTQD_RrEDUAvailBrkRgnTq_Nm) -> [VTQD_RrEDUAvailBrkRgnTq_Nm]
  Avaliable Torque/4(VTQD_FrRgnDecrSta_flg) -> [VTQD_FrRgnDecrSta_flg]
  Avaliable Torque/5(VTQD_RrRgnDecrSta_flg) -> [VTQD_RrRgnDecrSta_flg]
  Avaliable Torque/6(VTQD_FrRgnPermSta_flg) -> [VTQD_FrRgnPermSta_flg]
  Avaliable Torque/7(VTQD_RrRgnPermSta_flg) -> [VTQD_RrRgnPermSta_flg]
  [VTQD_DriverWhlTqDemFr_Nm] -> Bus Creator/9
  [VTQD_DriverWhlTqDemRr_Nm] -> Bus Creator/10
  [VTQD_ARegenActive_flg] -> Bus Creator/11
  [VTQD_FrEDUAvailBrkRgnTq_Nm] -> Bus Creator/12
  [VTQD_RrEDUAvailBrkRgnTq_Nm] -> Bus Creator/13
  [VTQD_FrRgnDecrSta_flg] -> Bus Creator/14
  [VTQD_RrRgnDecrSta_flg] -> Bus Creator/15
  [VTQD_FrRgnPermSta_flg] -> Bus Creator/16
  [VTQD_RrRgnPermSta_flg] -> Bus Creator/17
  [BSCPIn_outputs] -> ExtTqFuncHandShaking/1(BSCPIn_outputs)
  ExtTqFuncHandShaking/1(VTQD_ExternalTqAllow_flg) -> [VTQD_ExternalTqAllow_flg]
  ExtTqFuncHandShaking/2(VTQD_ExtShftAllow_flg) -> [VTQD_ExtShftAllow_flg]
  ExtTqFuncHandShaking/3(VTQD_ExtDoorAllow_flg) -> [VTQD_ExtDoorAllow_flg]
  [VTQD_ExternalTqAllow_flg] -> Bus Creator/18
  [VTQD_ExtShftAllow_flg] -> Bus Creator/19
  [VTQD_ExtDoorAllow_flg] -> Bus Creator/20
  [BSCPIn_outputs] -> Signal for ESC/1(BSCPIn_outputs)
  [BInpConvert_outputs] -> Signal for ESC/2(BInpConvert_outputs)
  [BMain_outputs] -> Signal for ESC/3(BMain_outputs)
  Signal for ESC/1(VTQD_FrEDUActTq_Nm) -> [VTQD_FrEDUActTq_Nm]
  Signal for ESC/2(VTQD_RrEDUActTq_Nm) -> [VTQD_RrEDUActTq_Nm]
  Signal for ESC/3(VTQD_FrEDURolRgnTq_Nm) -> [VTQD_FrEDURolRgnTq_Nm]
  Signal for ESC/4(VTQD_RrEDURolRgnTq_Nm) -> [VTQD_RrEDURolRgnTq_Nm]
  Signal for ESC/5(VTQD_FrEDUSpd_rpm) -> [VTQD_FrEDUSpd_rpm]
  Signal for ESC/6(VTQD_RrEDUSpd_rpm) -> [VTQD_RrEDUSpd_rpm]
  Signal for ESC/7(VTQD_FrEDUSpdValid_flg) -> [VTQD_FrEDUSpdValid_flg]
  Signal for ESC/8(VTQD_FrEDUActTqValid_flg) -> [VTQD_FrEDUActTqValid_flg]
  Signal for ESC/9(VTQD_FrEDURolRgnTqValid_flg) -> [VTQD_FrEDURolRgnTqValid_flg]
  Signal for ESC/10(VTQD_FrEDUAvailBrkRgnTqV_flg) -> [VTQD_FrEDUAvailBrkRgnTqV_flg]
  Signal for ESC/11(VTQD_RrEDUSpdValid_flg) -> [VTQD_RrEDUSpdValid_flg]
  Signal for ESC/12(VTQD_RrEDUActTqValid_flg) -> [VTQD_RrEDUActTqValid_flg]
  Signal for ESC/13(VTQD_RrEDURolRgnTqValid_flg) -> [VTQD_RrEDURolRgnTqValid_flg]
  Signal for ESC/14(VTQD_RrEDUAvailBrkRgnTqV_flg) -> [VTQD_RrEDUAvailBrkRgnTqV_flg]
  Signal for ESC/15(VTQD_RgnAbnorSta_flg) -> [VTQD_RgnAbnorSta_flg]
  Signal for ESC/16(VTQD_PTCSPermSta_flg) -> [VTQD_PTCSPermSta_flg]
  Signals for MCU/1(VTQD_FrIdcMin_A) -> [VTQD_FrIdcMin_A]
  Signals for MCU/2(VTQD_FrIdcMax_A) -> [VTQD_FrIdcMax_A]
  Signals for MCU/3(VTQD_FrUdcMin_V) -> [VTQD_FrUdcMin_V]
  Signals for MCU/4(VTQD_FrUdcMax_V) -> [VTQD_FrUdcMax_V]
  Signals for MCU/5(VTQD_RrIdcMin_A) -> [VTQD_RrIdcMin_A]
  Signals for MCU/6(VTQD_RrIdcMax_A) -> [VTQD_RrIdcMax_A]
  Signals for MCU/7(VTQD_RrUdcMin_V) -> [VTQD_RrUdcMin_V]
  Signals for MCU/8(VTQD_RrUdcMax_V) -> [VTQD_RrUdcMax_V]
  [BSCPIn_outputs] -> Signals for BCM/1(BSCPIn_outputs)
  [VTQD_ARegenActive_flg] -> Signals for BCM/2(VTQD_ARegenActive_flg)
  Signals for BCM/1(VTQD_ReBrakeLPReq_flg) -> [VTQD_ReBrakeLPReq_flg]
  [VTQD_FrEDUActTq_Nm] -> Bus Creator/21
  [VTQD_RrEDUActTq_Nm] -> Bus Creator/22
  [VTQD_FrEDURolRgnTq_Nm] -> Bus Creator/23
  [VTQD_RrEDURolRgnTq_Nm] -> Bus Creator/24
  [VTQD_FrEDUSpd_rpm] -> Bus Creator/25
  [VTQD_RrEDUSpd_rpm] -> Bus Creator/26
  [VTQD_FrEDUSpdValid_flg] -> Bus Creator/27  "VTQD_FrEDUSpdValid_flg"
  [VTQD_FrEDUActTqValid_flg] -> Bus Creator/28  "VTQD_FrEDUActTqValid_flg"
  [VTQD_FrEDURolRgnTqValid_flg] -> Bus Creator/29  "VTQD_FrEDURolRgnTqValid_flg"
  [VTQD_FrEDUAvailBrkRgnTqV_flg] -> Bus Creator/30
  [VTQD_RrEDUSpdValid_flg] -> Bus Creator/31  "VTQD_RrEDUSpdValid_flg"
  [VTQD_RrEDUActTqValid_flg] -> Bus Creator/32  "VTQD_RrEDUActTqValid_flg"
  [VTQD_RrEDURolRgnTqValid_flg] -> Bus Creator/33  "VTQD_RrEDURolRgnTqValid_flg"
  [VTQD_RrEDUAvailBrkRgnTqV_flg] -> Bus Creator/34
  [VTQD_RgnAbnorSta_flg] -> Bus Creator/35
  [VTQD_PTCSPermSta_flg] -> Bus Creator/36
  [VTQD_FrIdcMin_A] -> Bus Creator/37
  [VTQD_FrIdcMax_A] -> Bus Creator/38
  [VTQD_FrUdcMin_V] -> Bus Creator/39
  [VTQD_FrUdcMax_V] -> Bus Creator/40
  [VTQD_RrIdcMin_A] -> Bus Creator/41
  [VTQD_RrIdcMax_A] -> Bus Creator/42
  [VTQD_RrUdcMin_V] -> Bus Creator/43
  [VTQD_RrUdcMax_V] -> Bus Creator/44
  [VTQD_ReBrakeLPReq_flg] -> Bus Creator/45
  [BSCPIn_outputs] -> CrashDetect/1(BSCPIn_outputs)
  CrashDetect/1(VTQD_CrashDetd_flg) -> [VTQD_CrashDetd_flg]
  CrashDetect/2(VTQD_DiagHCrash_flg) -> [VTQD_DiagHCrash_flg]
  CrashDetect/3(VTQD_CrashUnlockReq_flg) -> [VTQD_CrashUnlockReq_flg]
  CrashDetect/4(VTQD_CTDCtrl_enum) -> [VTQD_CTDCtrl_enum]
  [VTQD_CrashUnlockReq_flg] -> Bus Creator/3
  [VTQD_CTDCtrl_enum] -> Bus Creator/4
